simulink model "sltestCruiseControlExample"  (R2018b)
settings: Solver=FixedStepDiscrete  StartTime=0.0  StopTime=1  FixedStep=0.01  RelTol=1e-3  EnableMultiTasking=on
PostLoadFcn:
  | load(fullfile(matlabroot,'examples','simulinktest','sltest_cruise_control_hierbus.mat'));
undefined symbols (not defined in the file or in its folder): DiscIntNeverNeededParam, sigbuilder_block, sldvsubsys
libraries: sldvlib x2
Description:
  | Defective Cruise Control
settings Model: Creator=The MathWorks, Inc.  LastModifiedBy=anjanak
settings DataIOCC: LimitDataPoints=on  SaveFormat=Array
settings OptimizationCC: ConditionallyExecuteInputs=off  DefaultParameterBehavior=Inlined  InlineInvariantSignals=on  ExpressionDepthLimit=2147483647  InitFltsAndDblsToZero=on  EfficientMapNaN2IntZero=off  LifeSpan=inf
settings DebuggingCC: SaveWithParameterizedLinksMsg=none  UnderspecifiedInitializationDetection=Classic  MergeDetectMultiDrivingBlocksExec=none  SignalResolutionControl=TryResolveAllWithWarning  SolverPrmCheckMsg=warning  FcnCallInpInsideContextMsg=warning  AllowSymbolicDim=off  StateNameClashWarn=warning  LibraryContextMissingDiagnostic=none  SFUnexpectedBacktrackingDiag=warning  SFNoUnconditionalDefaultTransitionDiag=warning  SFExecutionAtInitializationDiag=none
settings HardwareCC: ProdBitPerPointer=32  ProdBitPerSizeT=32  ProdBitPerPtrDiffT=32  ProdLargestAtomicFloat=None  ProdIntDivRoundTo=Undefined  ProdEndianess=Unspecified  ProdWordSize=32  ProdHWDeviceType=32-bit Generic
settings ModelReferenceCC: PropagateSignalLabelsOutOfModel=off
settings SFSimCC: SimUseLocalCustomCode=off
settings RTWCC: RTWUseLocalCustomCode=off
settings CodeAppCC: StateflowObjectComments=on
settings GRTTargetCC: TargetFcnLib=ansi_tfl_tmw.mat  TargetLangStandard=C89/C90 (ANSI)  GeneratePreprocessorConditionals=Disable all  CombineOutputUpdateFcns=off  GRTInterface=on
settings ConfigComp: CovMetricSettings=dcmse  DVMaxProcessTime=60  DVMakeOutputFilesUnique=off  DVParameters=on  DVModelCoverageObjectives=MCDC  DVMaxTestCaseSteps=500  DVTestSuiteOptimization=CombinedObjectives  DVAssertions=EnableAll  DVProofAssumptions=EnableAll  DVDetectActiveLogic=on  DVProvingStrategy=FindViolation

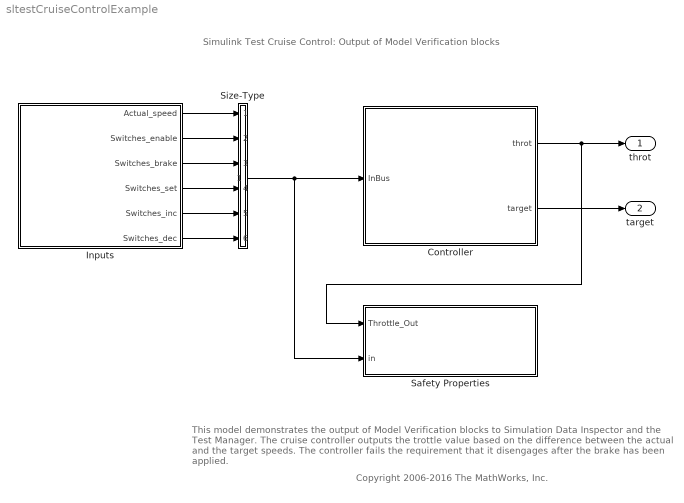
== system sltestCruiseControlExample ==
  note: Simulink Test Cruise Control: Output of Model Verification blocks
  note: Copyright 2006-2016 The MathWorks, Inc.
  note: This model demonstrates the output of Model Verification blocks to Simulation Data Inspector and the Test Manager. The cruise controller outputs the trottle value based on the difference between the actual and the target speeds. The controller fails the requirement that it disengages after the brake has been applied.
  Controller : Subsystem
  Inputs : Subsystem  Tag=STV Subsys  LoadFcn=sigbuilder_block('load');  StartFcn=sigbuilder_block('start');  StopFcn=sigbuilder_block('stop');  ClipboardFcn=sigbuilder_block('clipboard');  mask(Sigbuilder block){tuvar=[0:10]}
      mask init:
      | if ~strcmp(get_param(bdroot(gcb),'SimulationStatus'),'stopped'),tuvar = sigbuilder_block('maskInit'); end
      settings: CopyFcn=sigbuilder_block('copy');  DeleteFcn=sigbuilder_block('delete');  ModelCloseFcn=sigbuilder_block('modelClose');  PreSaveFcn=sigbuilder_block('preSave');  PauseFcn=sigbuilder_block('pause');  ContinueFcn=sigbuilder_block('continue');  NameChangeFcn=sigbuilder_block('namechange');  OpenFcn=sigbuilder_block('open',[171 169.5 519.75 474 ]);  CloseFcn=sigbuilder_block('close');
      mask Display: plot(0, 0, 100, 100,[2, 2, 32, 32, 2], [68, 8, 8, 68, 68],[32, 2], [38, 38], [32, 19, 2],[53, 60, 44], [32, 17, 17, 2],[16, 16, 31, 31]);txt = getActiveGroup(gcbh);text(2, 100, txt,'verticalAlignment', 'top');
  Safety Properties : Subsystem  Tag=VerificationSubsystem  DisableCoverage=on  LoadFcn=sldvsubsys('check')  TreatAsAtomicUnit=on  SimViewingDevice=on  mask(VerificationSubsystem){}
      mask init:
      | sldvsubsys('maskInit');
      settings: CopyFcn=sldvsubsys('copy');  OpenFcn=open_system(gcb,'force');
      settings: PreSaveFcn=|
      | set_param(gcb,'SimViewingDevice','on');
      | sldvsubsys('check');
      mask Help: helpview(fullfile(docroot,'toolbox','sldv','sldv.map'),'verificationsubsystem')
      mask Display: image(imread('sldvicon_versubsys.png','BackGroundColor',[1 1 1]),'center');
  Size-Type : Subsystem
  throt : Outport
  target : Outport  Port=2
  wires:
  Controller/2(target) -> target/1
  Inputs/1(Actual_speed) -> Size-Type/1(In1)
  Inputs/2(Switches_enable) -> Size-Type/2(In2)
  Inputs/3(Switches_brake) -> Size-Type/3(In3)
  Inputs/4(Switches_set) -> Size-Type/4(In4)
  Inputs/5(Switches_inc) -> Size-Type/5(In5)
  Inputs/6(Switches_dec) -> Size-Type/6(In6)
  Controller/1(throt) -> throt/1, Safety Properties/1(Throttle_Out)
  Size-Type/1(Out1) -> Safety Properties/2(in), Controller/1(InBus)

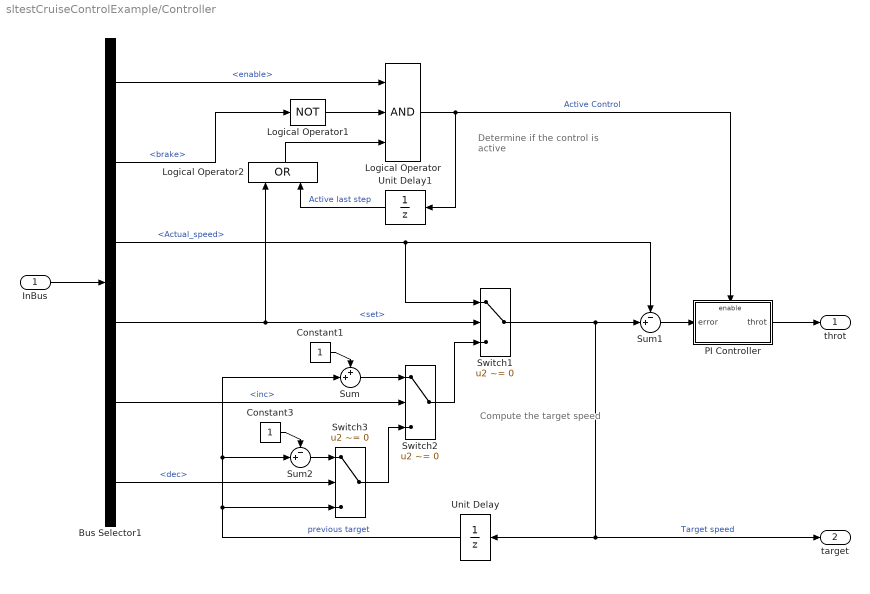
== system sltestCruiseControlExample/Controller ==
  note: Determine if the
      | control is active
  note: Compute the
      | target speed
  InBus : Inport  OutDataTypeStr=Bus: InputBus
  Bus Selector1 : BusSelector  OutputSignals=Switches.enable,Switches.brake,Actual_speed,Switches.set,Switches.setIncDec.inc,Switches.setIncDec.dec
  Constant1 : Constant
  Constant3 : Constant
  Logical Operator : Logic  Inputs=3  AllPortsSameDT=off  OutDataTypeStr=boolean
  Logical Operator1 : Logic  Operator=NOT  AllPortsSameDT=off  OutDataTypeStr=boolean
  Logical Operator2 : Logic  Operator=OR  AllPortsSameDT=off  OutDataTypeStr=boolean
  PI Controller : Subsystem
  Sum : Sum  Inputs=++|
  Sum1 : Sum  Inputs=-+|
  Sum2 : Sum  Inputs=-+|
  Switch1 : Switch  Criteria=u2 ~= 0
  Switch2 : Switch  Criteria=u2 ~= 0
  Switch3 : Switch  Criteria=u2 ~= 0
  Unit Delay : UnitDelay  SampleTime=0.01
  Unit Delay1 : UnitDelay  SampleTime=0.01
  throt : Outport
  target : Outport  Port=2
  wires:
  Logical Operator1/1 -> Logical Operator/2
  Constant1/1 -> Sum/1
  Sum/1 -> Switch2/1
  Constant3/1 -> Sum2/1
  Sum2/1 -> Switch3/1
  Switch2/1 -> Switch1/3
  Switch3/1 -> Switch2/3
  Unit Delay/1 -> Sum2/2, Sum/2, Switch3/3  "previous target"
  Switch1/1 -> Unit Delay/1, target/1, Sum1/2  "Target speed"
  Logical Operator2/1 -> Logical Operator/3
  Unit Delay1/1 -> Logical Operator2/2  "Active last step"
  Logical Operator/1 -> Unit Delay1/1, PI Controller/Enable  "Active Control"
  Sum1/1 -> PI Controller/1(error)
  InBus/1 -> Bus Selector1/1
  Bus Selector1/1 -> Logical Operator/1  "<enable>"
  Bus Selector1/2 -> Logical Operator1/1  "<brake>"
  Bus Selector1/4 -> Logical Operator2/1, Switch1/2  "<set>"
  Bus Selector1/5 -> Switch2/2  "<inc>"
  Bus Selector1/3 -> Sum1/1, Switch1/1  "<Actual_speed>"
  Bus Selector1/6 -> Switch3/2  "<dec>"
  PI Controller/1(throt) -> throt/1

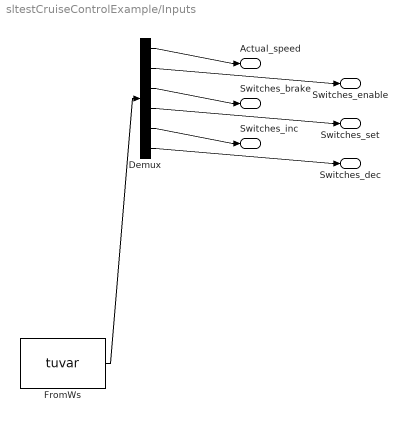
== system sltestCruiseControlExample/Inputs ==
  Demux : Demux  Tag=STV Demux  Outputs=6
  FromWs : FromWorkspace  Tag=STV FromWs  VariableName=tuvar  SampleTime=0
      SigBuilderData=|
      | dataSet.timeRange = [0 1]
      | dataSet.name = 'Sheet1'
      | sbobj.Name = 'Signal Builder'
      | sbobj.Groups.Name = 'Sheet1'
      | sbobj.Groups.Signals(1).Name = 'Actual_speed'
      | sbobj.Groups.Signals(1).XData = [0 0.01 0.02 0.03 0.04 0.05 0.06 0.07 0.08 0.09 0.1 0.11 0.12 0.13 0.14 0.15 0.16 0.17 0.18 0.19 0.2 0.21 0.22 0.23 0.24 0.25 0.26 0.27 0.28 0.29 0.3 0.31 0.32 0.33 0.34 0.35 0.36 0.37 0.38 0.39 0.4 0.41 0.42 0.43 0.44 0.45 0.46 0.47 0.48 0.49 0.5 0.51 0.52 0.53 0.54 0.55 0.56 0.57 0.58 0.59 0.6 0.61 0.62 0.63 0.64 0.65 0.66 0.67 0.68 0.69 0.7 0.71 0.72 0.73 0.74 0.75 0.76 0.77 0.78 0.79 0.8 0.81 0.82 0.83 0.84 0.85 0.86 0.87 0.88 0.89 0.9 0.91 0.92 0.93 0.94 0.95 0.96 0.97 0.98 0.99 1]
      | sbobj.Groups.Signals(1).YData = [40 40 40 40 40 40 40 40 40 40 40 40 40 40 40 40 40 40 40 40 40 40 40 40 40 40 40 40 40 40 40 40 40 40 40 40 40 40 40 40 40 40 40 40 40 40 40 40 40 40 40 40 40 40 40 40 40 40 40 40 40 40 40 40 40 40 40 40 40 40 40 40 40 40 40 40 40 40 40 40 40 40 40 40 40 40 40 40 40 40 40 40 40 40 40 40 40 40 40 40 40]
      | sbobj.Groups.Signals(2).Name = 'Switches_enable'
      | sbobj.Groups.Signals(2).XData = [0 0.01 0.02 0.03 0.04 0.05 0.06 0.07 0.08 0.09 0.1 0.11 0.12 0.13 0.14 0.15 0.16 0.17 0.18 0.19 0.2 0.21 0.22 0.23 0.24 0.25 0.26 0.27 0.28 0.29 0.3 0.31 0.32 0.33 0.34 0.35 0.36 0.37 0.38 0.39 0.4 0.41 0.42 0.43 0.44 0.45 0.46 0.47 0.48 0.49 0.5 0.51 0.52 0.53 0.54 0.55 0.56 0.57 0.58 0.59 0.6 0.61 0.62 0.63 0.64 0.65 0.66 0.67 0.68 0.69 0.7 0.71 0.72 0.73 0.74 0.75 0.76 0.77 0.78 0.79 0.8 0.81 0.82 0.83 0.84 0.85 0.86 0.87 0.88 0.89 0.9 0.91 0.92 0.93 0.94 0.95 0.96 0.97 0.98 0.99 1]
      | sbobj.Groups.Signals(2).YData = [1 1 1 1 1 1 1 1 1 1 1 1 1 1 1 1 1 1 1 1 1 1 1 1 1 1 1 1 1 1 1 1 1 1 1 1 1 1 1 1 1 1 1 1 1 1 1 1 1 1 1 1 1 1 1 1 1 1 1 1 1 1 1 1 1 1 1 1 1 1 1 1 1 1 1 1 1 1 1 1 1 1 1 1 1 1 1 1 1 1 1 1 1 1 1 1 1 1 1 1 1]
      | sbobj.Groups.Signals(3).Name = 'Switches_brake'
      | sbobj.Groups.Signals(3).XData = [0 0.01 0.02 0.03 0.04 0.05 0.06 0.07 0.08 0.09 0.1 0.11 0.12 0.13 0.14 0.15 0.16 0.17 0.18 0.19 0.2 0.21 0.22 0.23 0.24 0.25 0.26 0.27 0.28 0.29 0.3 0.31 0.32 0.33 0.34 0.35 0.36 0.37 0.38 0.39 0.4 0.41 0.42 0.43 0.44 0.45 0.46 0.47 0.48 0.49 0.5 0.51 0.52 0.53 0.54 0.55 0.56 0.57 0.58 0.59 0.6 0.61 0.62 0.63 0.64 0.65 0.66 0.67 0.68 0.69 0.7 0.71 0.72 0.73 0.74 0.75 0.76 0.77 0.78 0.79 0.8 0.81 0.82 0.83 0.84 0.85 0.86 0.87 0.88 0.89 0.9 0.91 0.92 0.93 0.94 0.95 0.96 0.97 0.98 0.99 1]
      | sbobj.Groups.Signals(3).YData = [0 0 0 0 0 0 0 0 0 0 0 0 0 0 0 0 0 0 0 0 0 1 1 1 1 1 1 1 1 1 1 1 1 1 1 1 1 1 1 1 1 1 1 1 1 1 1 1 1 1 1 1 1 1 1 1 1 1 1 1 1 1 1 1 1 1 1 1 1 1 1 1 1 1 1 1 1 1 1 1 1 1 1 1 1 1 1 1 1 1 1 1 1 1 1 1 1 1 1 1 1]
      | sbobj.Groups.Signals(4).Name = 'Switches_set'
      | sbobj.Groups.Signals(4).XData = [0 0.01 0.02 0.03 0.04 0.05 0.06 0.07 0.08 0.09 0.1 0.11 0.12 0.13 0.14 0.15 0.16 0.17 0.18 0.19 0.2 0.21 0.22 0.23 0.24 0.25 0.26 0.27 0.28 0.29 0.3 0.31 0.32 0.33 0.34 0.35 0.36 0.37 0.38 0.39 0.4 0.41 0.42 0.43 0.44 0.45 0.46 0.47 0.48 0.49 0.5 0.51 0.52 0.53 0.54 0.55 0.56 0.57 0.58 0.59 0.6 0.61 0.62 0.63 0.64 0.65 0.66 0.67 0.68 0.69 0.7 0.71 0.72 0.73 0.74 0.75 0.76 0.77 0.78 0.79 0.8 0.81 0.82 0.83 0.84 0.85 0.86 0.87 0.88 0.89 0.9 0.91 0.92 0.93 0.94 0.95 0.96 0.97 0.98 0.99 1]
      | sbobj.Groups.Signals(4).YData = [1 1 0 0 0 0 0 0 0 0 0 0 0 0 0 0 0 0 0 0 0 0 0 0 0 0 0 0 0 0 0 0 0 0 0 0 0 0 0 0 0 0 0 0 0 0 0 0 0 0 0 0 0 0 0 0 0 0 0 0 0 0 0 0 0 0 0 0 0 0 0 0 0 0 0 0 0 0 0 0 0 0 0 0 0 0 0 0 0 0 0 0 0 0 0 0 0 0 0 0 0]
      | sbobj.Groups.Signals(5).Name = 'Switches_inc'
      | sbobj.Groups.Signals(5).XData = [0 0.01 0.02 0.03 0.04 0.05 0.06 0.07 0.08 0.09 0.1 0.11 0.12 0.13 0.14 0.15 0.16 0.17 0.18 0.19 0.2 0.21 0.22 0.23 0.24 0.25 0.26 0.27 0.28 0.29 0.3 0.31 0.32 0.33 0.34 0.35 0.36 0.37 0.38 0.39 0.4 0.41 0.42 0.43 0.44 0.45 0.46 0.47 0.48 0.49 0.5 0.51 0.52 0.53 0.54 0.55 0.56 0.57 0.58 0.59 0.6 0.61 0.62 0.63 0.64 0.65 0.66 0.67 0.68 0.69 0.7 0.71 0.72 0.73 0.74 0.75 0.76 0.77 0.78 0.79 0.8 0.81 0.82 0.83 0.84 0.85 0.86 0.87 0.88 0.89 0.9 0.91 0.92 0.93 0.94 0.95 0.96 0.97 0.98 0.99 1]
      | sbobj.Groups.Signals(5).YData = [1 1 1 0 0 0 0 0 0 0 0 0 0 0 0 0 0 0 0 0 0 0 0 0 0 0 0 0 0 0 0 0 0 0 0 0 0 0 0 0 0 0 0 0 0 0 0 0 0 0 0 0 0 0 0 0 0 0 0 0 0 0 0 0 0 0 0 0 0 0 0 0 0 0 0 0 0 0 0 0 0 0 0 0 0 0 0 0 0 0 0 0 0 0 0 0 0 0 0 0 0]
      | sbobj.Groups.Signals(6).Name = 'Switches_dec'
      | sbobj.Groups.Signals(6).XData = [0 0.01 0.02 0.03 0.04 0.05 0.06 0.07 0.08 0.09 0.1 0.11 0.12 0.13 0.14 0.15 0.16 0.17 0.18 0.19 0.2 0.21 0.22 0.23 0.24 0.25 0.26 0.27 0.28 0.29 0.3 0.31 0.32 0.33 0.34 0.35 0.36 0.37 0.38 0.39 0.4 0.41 0.42 0.43 0.44 0.45 0.46 0.47 0.48 0.49 0.5 0.51 0.52 0.53 0.54 0.55 0.56 0.57 0.58 0.59 0.6 0.61 0.62 0.63 0.64 0.65 0.66 0.67 0.68 0.69 0.7 0.71 0.72 0.73 0.74 0.75 0.76 0.77 0.78 0.79 0.8 0.81 0.82 0.83 0.84 0.85 0.86 0.87 0.88 0.89 0.9 0.91 0.92 0.93 0.94 0.95 0.96 0.97 0.98 0.99 1]
      | sbobj.Groups.Signals(6).YData = [0 0 0 0 0 0 0 0 0 0 0 0 0 0 0 0 0 0 0 0 0 0 0 0 0 0 0 0 0 0 0 0 0 0 0 0 0 0 0 0 0 0 0 0 0 0 0 0 0 0 0 0 0 0 0 0 0 0 0 0 0 0 0 0 0 0 0 0 0 0 0 0 0 0 0 0 0 0 0 0 0 0 0 0 0 0 0 0 0 0 0 0 0 0 0 0 0 0 0 0 0]
      | sbobj.Groups.TimeRange = [0 1]
  Actual_speed : Outport  Tag=STV Outport
  Switches_enable : Outport  Tag=STV Outport  Port=2
  Switches_brake : Outport  Tag=STV Outport  Port=3
  Switches_set : Outport  Tag=STV Outport  Port=4
  Switches_inc : Outport  Tag=STV Outport  Port=5
  Switches_dec : Outport  Tag=STV Outport  Port=6
  wires:
  FromWs/1 -> Demux/1
  Demux/1 -> Actual_speed/1
  Demux/2 -> Switches_enable/1
  Demux/3 -> Switches_brake/1
  Demux/4 -> Switches_set/1
  Demux/5 -> Switches_inc/1
  Demux/6 -> Switches_dec/1

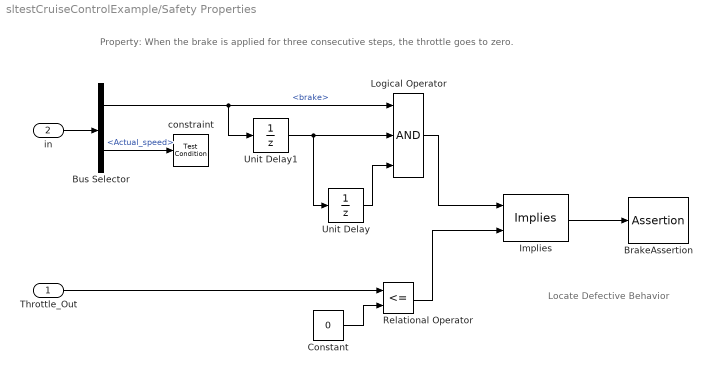
== system sltestCruiseControlExample/Safety Properties ==
  note: Property: When the brake is applied for three consecutive steps, the throttle goes to zero.
  note: Locate Defective Behavior
  Throttle_Out : Inport
  in : Inport  Port=2  OutDataTypeStr=Bus: InputBus
  BrakeAssertion : Assertion  StopWhenAssertionFail=off
  Bus Selector : BusSelector  OutputSignals=Switches.brake,Actual_speed
  Constant : Constant  Value=0
  Implies : sldvlib/Verification Utilities/Implies
      settings: SourceProductName=Simulink Design Verifier  SourceProductBaseCode=DV
  Logical Operator : Logic  Inputs=3  AllPortsSameDT=off  OutDataTypeStr=boolean
  Relational Operator : RelationalOperator  Operator=<=  OutDataTypeStr=boolean  RndMeth=Nearest
  Unit Delay : UnitDelay  SampleTime=-1
  Unit Delay1 : UnitDelay  SampleTime=-1
  constraint : sldvlib/Objectives and Constraints/Test Condition  enabled=on  customAVTBlockType=Assumption  intervals=[0 100]  initial=off  dispValues=on  outEnabled=off
      settings: AttributesFormatString=%<intervals>  SourceProductName=Simulink Design Verifier  SourceProductBaseCode=DV
  wires:
  Bus Selector/1 -> Unit Delay1/1, Logical Operator/1  "<brake>"
  Unit Delay1/1 -> Unit Delay/1, Logical Operator/2
  Unit Delay/1 -> Logical Operator/3
  Logical Operator/1 -> Implies/1
  Implies/1 -> BrakeAssertion/1
  Constant/1 -> Relational Operator/2
  Relational Operator/1 -> Implies/2
  in/1 -> Bus Selector/1
  Bus Selector/2 -> constraint/1  "<Actual_speed>"
  Throttle_Out/1 -> Relational Operator/1

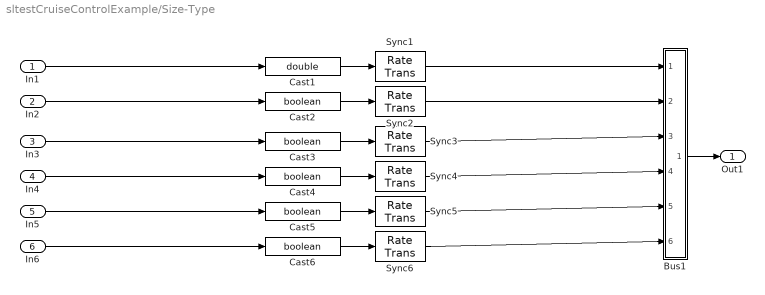
== system sltestCruiseControlExample/Size-Type ==
  In1 : Inport
  In2 : Inport  Port=2
  In3 : Inport  Port=3
  In4 : Inport  Port=4
  In5 : Inport  Port=5
  In6 : Inport  Port=6
  Bus1 : Subsystem
  Cast1 : DataTypeConversion  OutDataTypeStr=double  RndMeth=Nearest  SaturateOnIntegerOverflow=on
  Cast{2..6} (5 alike) : DataTypeConversion  OutDataTypeStr=boolean  RndMeth=Nearest  SaturateOnIntegerOverflow=on
  Sync{1..6} (6 alike) : RateTransition  OutPortSampleTime=[0.01,0]
  Out1 : Outport
  wires:
  In1/1 -> Cast1/1
  Cast1/1 -> Sync1/1
  In2/1 -> Cast2/1
  Cast2/1 -> Sync2/1
  In3/1 -> Cast3/1
  Cast3/1 -> Sync3/1
  In4/1 -> Cast4/1
  Cast4/1 -> Sync4/1
  In5/1 -> Cast5/1
  Cast5/1 -> Sync5/1
  In6/1 -> Cast6/1
  Cast6/1 -> Sync6/1
  Sync1/1 -> Bus1/1(InputData(1).Actual_speed)
  Sync2/1 -> Bus1/2(InputData(1).Switches(1).enable)
  Sync3/1 -> Bus1/3(InputData(1).Switches(1).brake)
  Sync4/1 -> Bus1/4(InputData(1).Switches(1).set)
  Sync5/1 -> Bus1/5(InputData(1).Switches(1).setIncDec(1).inc)
  Sync6/1 -> Bus1/6(InputData(1).Switches(1).setIncDec(1).dec)
  Bus1/1(Out) -> Out1/1

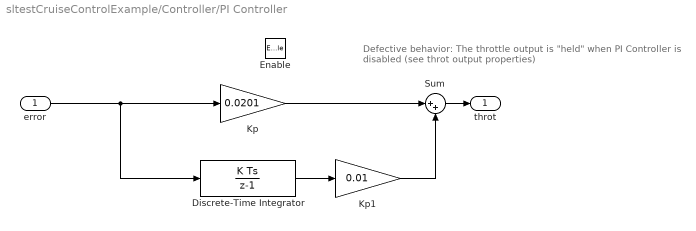
== system sltestCruiseControlExample/Controller/PI Controller ==
  note: Defective behavior: The throttle output is "held" when
      | PI Controller is disabled (see throt output properties)
  error : Inport
  Enable : EnablePort  PropagateVarSize=During execution
  Discrete-Time Integrator : DiscreteIntegrator  SampleTime=0.01  LimitOutput=on  UpperSaturationLimit=5  LowerSaturationLimit=-5  ICPrevOutput=DiscIntNeverNeededParam  ICPrevScaledInput=DiscIntNeverNeededParam
  Kp : Gain  Gain=0.0201
  Kp1 : Gain  Gain=0.01
  Sum : Sum  Inputs=|++
  throt : Outport  OutputWhenDisabled=reset  InitialOutput=0
  wires:
  Kp/1 -> Sum/1
  Kp1/1 -> Sum/2
  Discrete-Time Integrator/1 -> Kp1/1
  error/1 -> Kp/1, Discrete-Time Integrator/1
  Sum/1 -> throt/1

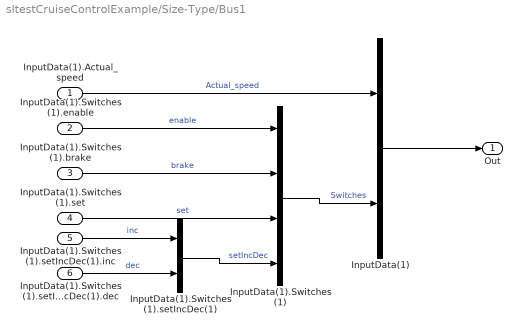
== system sltestCruiseControlExample/Size-Type/Bus1 ==
  InputData(1).Actual_speed : Inport
  InputData(1).Switches(1).enable : Inport  Port=2
  InputData(1).Switches(1).brake : Inport  Port=3
  InputData(1).Switches(1).set : Inport  Port=4
  InputData(1).Switches(1).setIncDec(1).inc : Inport  Port=5
  InputData(1).Switches(1).setIncDec(1).dec : Inport  Port=6
  InputData(1) : BusCreator  Inputs=2  OutDataTypeStr=Bus: InputBus  NonVirtualBus=on
  InputData(1).Switches(1) : BusCreator  Inputs=4  OutDataTypeStr=Bus: Switches  NonVirtualBus=on
  InputData(1).Switches(1).setIncDec(1) : BusCreator  Inputs=2  OutDataTypeStr=Bus: setpoint  NonVirtualBus=on
  Out : Outport
  wires:
  InputData(1).Switches(1).setIncDec(1).inc/1 -> InputData(1).Switches(1).setIncDec(1)/1  "inc"
  InputData(1).Switches(1).setIncDec(1).dec/1 -> InputData(1).Switches(1).setIncDec(1)/2  "dec"
  InputData(1).Switches(1).enable/1 -> InputData(1).Switches(1)/1  "enable"
  InputData(1).Switches(1).brake/1 -> InputData(1).Switches(1)/2  "brake"
  InputData(1).Switches(1).set/1 -> InputData(1).Switches(1)/3  "set"
  InputData(1).Switches(1).setIncDec(1)/1 -> InputData(1).Switches(1)/4  "setIncDec"
  InputData(1).Actual_speed/1 -> InputData(1)/1  "Actual_speed"
  InputData(1).Switches(1)/1 -> InputData(1)/2  "Switches"
  InputData(1)/1 -> Out/1
